simulink model "simple_hearing_aid"  (R2020b)
settings: Solver=FixedStepDiscrete  StartTime=0.0  StopTime=stopTime  RelTol=1e-3
PreLoadFcn:
  | addpath(genpath('..\fast_fourier_transform'));
  | addpath(genpath('..\fft_filters'));
  | addpath(genpath('..\noise_suppression'));
InitFcn:
  | initCallback
StopFcn:
  | stopCallback
undefined symbols (not defined in the file or in its folder): config, mp
settings Model: Creator=Ross  LastModifiedBy=conno
settings SolverCC: AutoInsertRateTranBlk=on
settings DataIOCC: ReturnWorkspaceOutputs=off
settings OptimizationCC: BlockReduction=off  ConditionallyExecuteInputs=off  DefaultParameterBehavior=Inlined
settings DebuggingCC: SignalInfNanChecking=error  SignalRangeChecking=warning  ReadBeforeWriteMsg=DisableAll  WriteAfterWriteMsg=DisableAll  WriteAfterReadMsg=DisableAll  AlgebraicLoopMsg=error  MultiTaskDSMMsg=none  SingleTaskRateTransMsg=error  ParameterUnderflowMsg=warning  UnderSpecifiedDataTypeMsg=error  PregeneratedLibrarySubsystemCodeDiagnostic=none  ArithmeticOperatorsInVariantConditions=warning
settings HardwareCC: ProdBitPerPointer=32  ProdBitPerSizeT=32  ProdBitPerPtrDiffT=32  ProdLargestAtomicFloat=None  ProdIntDivRoundTo=Undefined  ProdEndianess=Unspecified  ProdWordSize=32  ProdHWDeviceType=ASIC/FPGA->ASIC/FPGA  TargetBitPerPointer=64  TargetBitPerSizeT=64  TargetBitPerPtrDiffT=64  TargetLongLongMode=on  TargetIntDivRoundTo=Zero  TargetEndianess=LittleEndian  TargetWordSize=64  TargetHWDeviceType=Custom Processor->MATLAB Host Computer  ProdEqTarget=off
settings ModelReferenceCC: UpdateModelReferenceTargets=IfOutOfDate
settings SFSimCC: SFSimEcho=off  SimUseLocalCustomCode=off  CustomCodeUndefinedFunction=UseInterfaceOnly
settings RTWCC: RTWUseLocalCustomCode=off

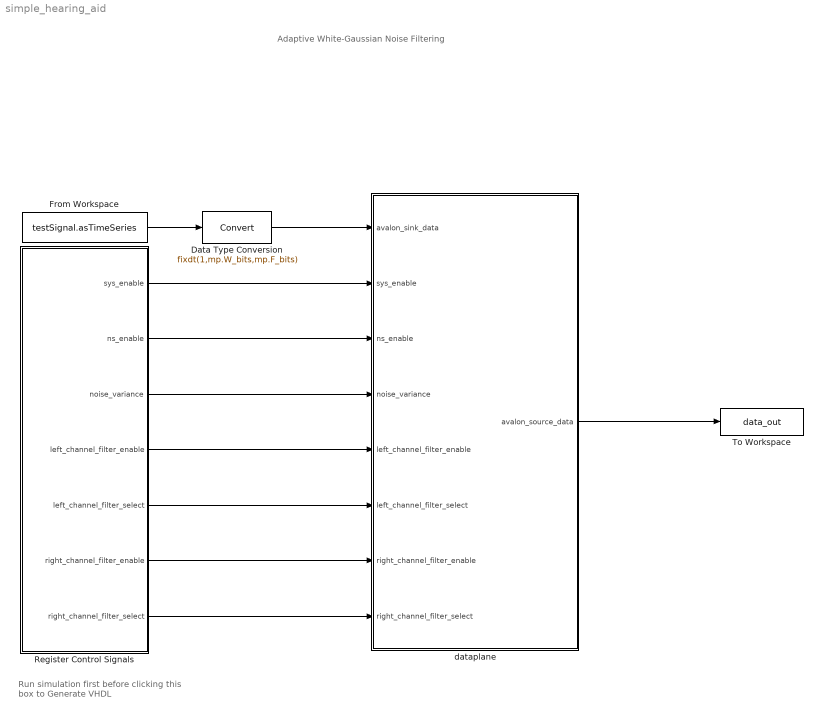
== system simple_hearing_aid ==
  note: Adaptive White-Gaussian Noise Filtering
  note: Run simulation first
      | before clicking this box to
      | Generate VHDL
  Data Type Conversion : DataTypeConversion  OutDataTypeStr=fixdt(1,mp.W_bits,mp.F_bits)
  From Workspace : FromWorkspace  VariableName=testSignal.asTimeSeries  OutDataTypeStr=double  SampleTime=1 / config.system.sampleClockFrequency  Interpolate=off  OutputAfterFinalValue=Setting to zero
  Register Control Signals : Subsystem
  To Workspace : ToWorkspace  VariableName=data_out  SampleTime=-1
      settings: Save2DSignal=2-D array (concatenate along first dimension)
  dataplane : Subsystem  TreatAsAtomicUnit=on
  wires:
  dataplane/1(avalon_source_data) -> To Workspace/1
  From Workspace/1 -> Data Type Conversion/1
  Data Type Conversion/1 -> dataplane/1(avalon_sink_data)
  Register Control Signals/5(left_channel_filter_select) -> dataplane/6(left_channel_filter_select)
  Register Control Signals/4(left_channel_filter_enable) -> dataplane/5(left_channel_filter_enable)
  Register Control Signals/3(noise_variance) -> dataplane/4(noise_variance)
  Register Control Signals/2(ns_enable) -> dataplane/3(ns_enable)
  Register Control Signals/1(sys_enable) -> dataplane/2(sys_enable)
  Register Control Signals/6(right_channel_filter_enable) -> dataplane/7(right_channel_filter_enable)
  Register Control Signals/7(right_channel_filter_select) -> dataplane/8(right_channel_filter_select)

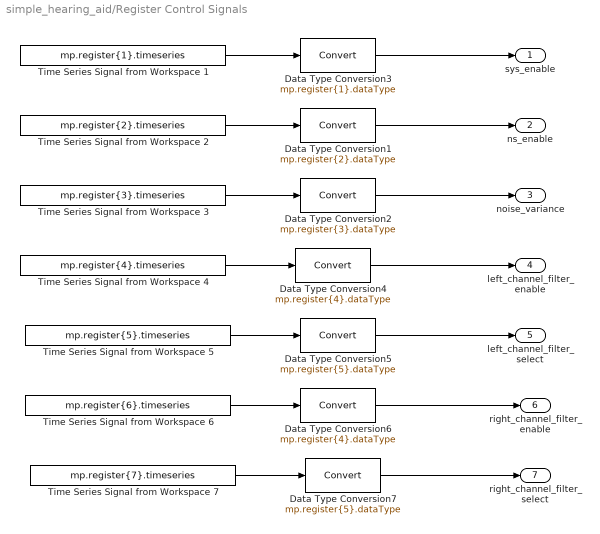
== system simple_hearing_aid/Register Control Signals ==
  Data Type Conversion1 : DataTypeConversion  OutDataTypeStr=mp.register{2}.dataType
  Data Type Conversion2 : DataTypeConversion  OutDataTypeStr=mp.register{3}.dataType
  Data Type Conversion3 : DataTypeConversion  OutDataTypeStr=mp.register{1}.dataType
  Data Type Conversion4 : DataTypeConversion  OutDataTypeStr=mp.register{4}.dataType
  Data Type Conversion5 : DataTypeConversion  OutDataTypeStr=mp.register{5}.dataType
  Data Type Conversion6 : DataTypeConversion  OutDataTypeStr=mp.register{4}.dataType
  Data Type Conversion7 : DataTypeConversion  OutDataTypeStr=mp.register{5}.dataType
  Time Series Signal from Workspace 1 : FromWorkspace  VariableName=mp.register{1}.timeseries  OutDataTypeStr=double  SampleTime=1 / config.system.sampleClockFrequency
  Time Series Signal from Workspace 2 : FromWorkspace  VariableName=mp.register{2}.timeseries  OutDataTypeStr=double  SampleTime=1 / config.system.sampleClockFrequency
  Time Series Signal from Workspace 3 : FromWorkspace  VariableName=mp.register{3}.timeseries  OutDataTypeStr=double  SampleTime=1 / config.system.sampleClockFrequency
  Time Series Signal from Workspace 4 : FromWorkspace  VariableName=mp.register{4}.timeseries  OutDataTypeStr=double  SampleTime=1 / config.system.sampleClockFrequency
  Time Series Signal from Workspace 5 : FromWorkspace  VariableName=mp.register{5}.timeseries  OutDataTypeStr=double  SampleTime=1 / config.system.sampleClockFrequency
  Time Series Signal from Workspace 6 : FromWorkspace  VariableName=mp.register{6}.timeseries  OutDataTypeStr=double  SampleTime=1 / config.system.sampleClockFrequency
  Time Series Signal from Workspace 7 : FromWorkspace  VariableName=mp.register{7}.timeseries  OutDataTypeStr=double  SampleTime=1 / config.system.sampleClockFrequency
  sys_enable : Outport  VectorParamsAs1DForOutWhenUnconnected=off
  ns_enable : Outport  Port=2  VectorParamsAs1DForOutWhenUnconnected=off
  noise_variance : Outport  Port=3  VectorParamsAs1DForOutWhenUnconnected=off
  left_channel_filter_enable : Outport  Port=4  VectorParamsAs1DForOutWhenUnconnected=off
  left_channel_filter_select : Outport  Port=5  VectorParamsAs1DForOutWhenUnconnected=off
  right_channel_filter_enable : Outport  Port=6  VectorParamsAs1DForOutWhenUnconnected=off
  right_channel_filter_select : Outport  Port=7  VectorParamsAs1DForOutWhenUnconnected=off
  wires:
  Data Type Conversion1/1 -> ns_enable/1
  Data Type Conversion2/1 -> noise_variance/1
  Data Type Conversion3/1 -> sys_enable/1
  Data Type Conversion4/1 -> left_channel_filter_enable/1
  Time Series Signal from Workspace 4/1 -> Data Type Conversion4/1
  Time Series Signal from Workspace 2/1 -> Data Type Conversion1/1
  Time Series Signal from Workspace 1/1 -> Data Type Conversion3/1
  Time Series Signal from Workspace 3/1 -> Data Type Conversion2/1
  Time Series Signal from Workspace 5/1 -> Data Type Conversion5/1
  Data Type Conversion5/1 -> left_channel_filter_select/1
  Time Series Signal from Workspace 6/1 -> Data Type Conversion6/1
  Time Series Signal from Workspace 7/1 -> Data Type Conversion7/1
  Data Type Conversion7/1 -> right_channel_filter_select/1
  Data Type Conversion6/1 -> right_channel_filter_enable/1

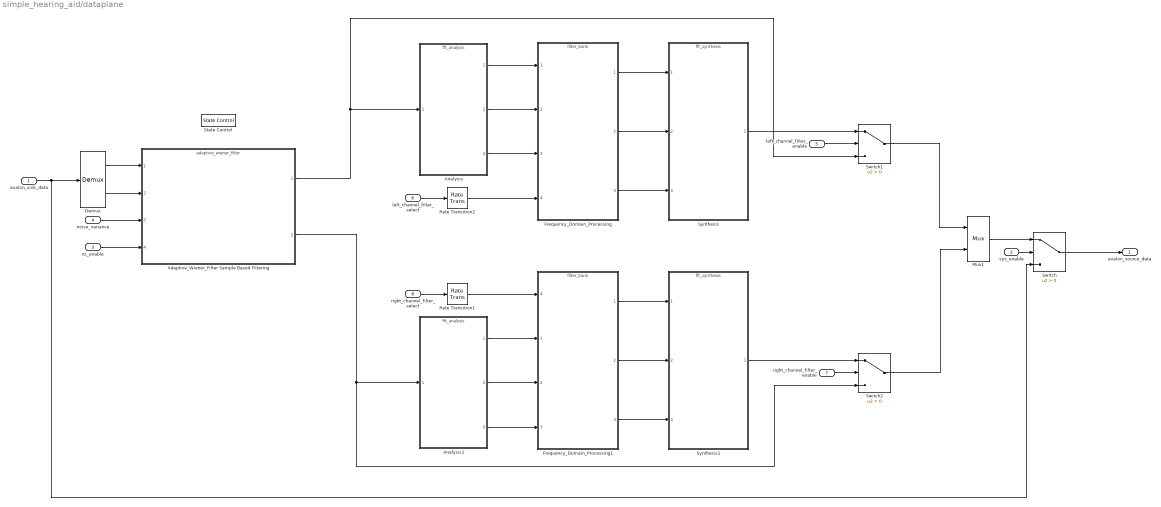
== system simple_hearing_aid/dataplane ==
  avalon_sink_data : Inport
  sys_enable : Inport  Port=2
  ns_enable : Inport  Port=3
  noise_variance : Inport  Port=4
  left_channel_filter_enable : Inport  Port=5
  left_channel_filter_select : Inport  Port=6
  right_channel_filter_enable : Inport  Port=7
  right_channel_filter_select : Inport  Port=8
  Adaptive_Wiener_Filter Sample Based Filtering : ModelReference  ModelNameDialog=adaptive_wiener_filter  SimulationMode=Normal  ModelReferenceVersion=2.6
  Analysis : ModelReference  ModelNameDialog=fft_analysis  SimulationMode=Normal  ModelReferenceVersion=1.151
  Analysis1 : ModelReference  ModelNameDialog=fft_analysis  SimulationMode=Normal  ModelReferenceVersion=1.151
  Demux : Demux  Outputs=2
      settings: DisplayOption=none
  Frequency_Domain_Processing : ModelReference  ModelNameDialog=filter_bank  SimulationMode=Normal  ModelReferenceVersion=1.142
  Frequency_Domain_Processing1 : ModelReference  ModelNameDialog=filter_bank  SimulationMode=Normal  ModelReferenceVersion=1.142
      settings: PortSchema="{\"entries\":[{\"content\":{\"sides\":[{\"content\":{\"connectorIds\":[\"In4\",\"In1\",\"In2\",\"In3\"]},\"type\":\"ConnectorPlacement.EquallySpacedRectSide\",\"uuid\":\"98b9ab6b-e920-433b-8eaa-544dbbe55daf\"},{\"content\":{\"connectorIds\":[\"Out1\",\"Out2\",\"Out3\"],\"side\":\"RIGHT\"},\"type\":\"ConnectorPlacement.EquallySpacedRectSide\",\"uuid\":\"23afa30c-ea88-4878-82e5-93b2404d6220\"},{\"content\":{\"connectorIds\":[],\"side\":\"TOP\"},\"type\":\"ConnectorPlacement.EquallySpacedRectSide\",\"uuid\":\"150f35b0-e320-4333-af3d-b6ee6411669e\"},{\"content\":{\"connectorIds\":[],\"side\":\"HIDDEN\"},\"type\":\"ConnectorPlacement.EquallySpacedRectSide\",\"uuid\":\"5a87abe7-f104-42bf-9aca-dc77348fd7fe\"}]},\"type\":\"ConnectorPlacement.EquallySpacedConnector\",\"uuid\":\"00b47f52-c791-4962-ab7a-975dce87c70e\"}],\"packageUris\":[\"http://schema.mathworks.com/mf0/Connector/R2020b\"],\"version\":\"1.0\"}"
  Mux1 : Mux  Inputs=2
  Rate Transition1 : RateTransition  InitialCondition=3  OutPortSampleTimeOpt=Multiple of input port sample time  OutPortSampleTimeMultiple=1/mp.SysRate_Upsample_Factor
  Rate Transition2 : RateTransition  InitialCondition=3  OutPortSampleTimeOpt=Multiple of input port sample time  OutPortSampleTimeMultiple=1/mp.SysRate_Upsample_Factor
  State Control : StateControl  StateControl=Synchronous
  Switch : Switch  Criteria=u2 > Threshold
  Switch1 : Switch  Criteria=u2 > Threshold
  Switch2 : Switch  Criteria=u2 > Threshold
  Synthesis : ModelReference  ModelNameDialog=fft_synthesis.slx  SimulationMode=Normal  ModelReferenceVersion=3.10
  Synthesis1 : ModelReference  ModelNameDialog=fft_synthesis.slx  SimulationMode=Normal  ModelReferenceVersion=3.10
  avalon_source_data : Outport  VectorParamsAs1DForOutWhenUnconnected=off
  wires:
  noise_variance/1 -> Adaptive_Wiener_Filter Sample Based Filtering/3
  Demux/2 -> Adaptive_Wiener_Filter Sample Based Filtering/2
  Demux/1 -> Adaptive_Wiener_Filter Sample Based Filtering/1
  avalon_sink_data/1 -> Switch/3, Demux/1
  Switch/1 -> avalon_source_data/1
  ns_enable/1 -> Adaptive_Wiener_Filter Sample Based Filtering/4
  Frequency_Domain_Processing/1 -> Synthesis/1
  Adaptive_Wiener_Filter Sample Based Filtering/1 -> Analysis/1, Switch1/3
  Analysis/3 -> Frequency_Domain_Processing/3
  Frequency_Domain_Processing/2 -> Synthesis/2
  Analysis/2 -> Frequency_Domain_Processing/2
  Rate Transition2/1 -> Frequency_Domain_Processing/4
  Frequency_Domain_Processing/3 -> Synthesis/3
  Analysis/1 -> Frequency_Domain_Processing/1
  left_channel_filter_select/1 -> Rate Transition2/1
  Frequency_Domain_Processing1/1 -> Synthesis1/1
  Adaptive_Wiener_Filter Sample Based Filtering/2 -> Switch2/3, Analysis1/1
  Analysis1/3 -> Frequency_Domain_Processing1/3
  Frequency_Domain_Processing1/2 -> Synthesis1/2
  Analysis1/2 -> Frequency_Domain_Processing1/2
  Frequency_Domain_Processing1/3 -> Synthesis1/3
  Analysis1/1 -> Frequency_Domain_Processing1/1
  Mux1/1 -> Switch/1
  sys_enable/1 -> Switch/2
  Synthesis/1 -> Switch1/1
  Switch1/1 -> Mux1/1
  Synthesis1/1 -> Switch2/1
  Switch2/1 -> Mux1/2
  left_channel_filter_enable/1 -> Switch1/2
  right_channel_filter_select/1 -> Rate Transition1/1
  Rate Transition1/1 -> Frequency_Domain_Processing1/4
  right_channel_filter_enable/1 -> Switch2/2
